simulink model "Enable_Subsystem_Step"  (R2024b)
settings: Solver=FixedStepAuto  StartTime=0.0  StopTime=10.0  FixedStep=0.001  RelTol=1e-3
settings Model: Creator=abdal  LastModifiedBy=abdal

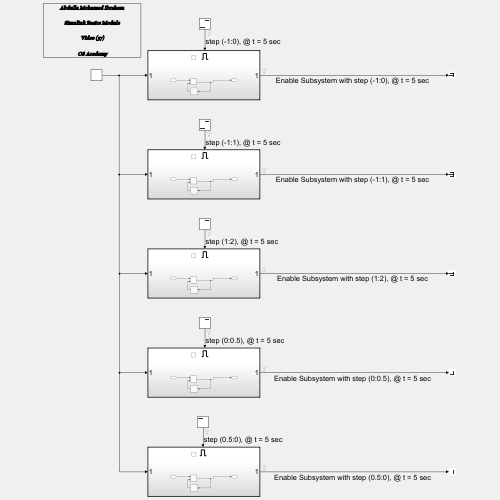
[thumbnail: Simulink's stored preview of the top-level diagram]
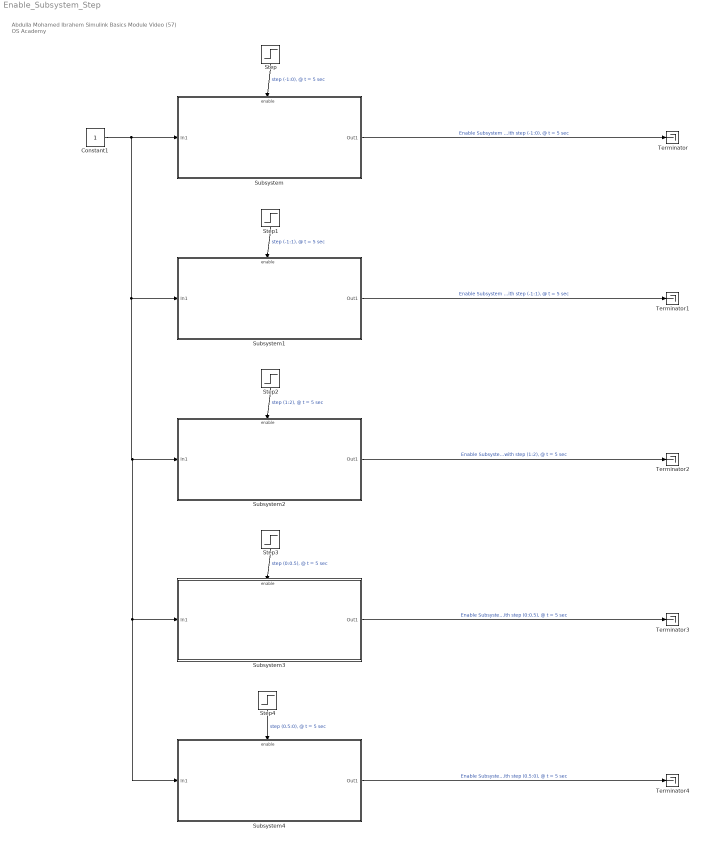
== system Enable_Subsystem_Step ==
  note: Abdulla Mohamed Ibrahem
      | Simulink Basics Module
      | Video (57)
      | OS Academy
  Constant1 : Constant
  Step : Step  Time=5  Before=-1  After=0  SampleTime=0
  Step1 : Step  Time=5  Before=-1  SampleTime=0
  Step2 : Step  Time=5  Before=1  After=2  SampleTime=0
  Step3 : Step  Time=5  After=0.5  SampleTime=0
  Step4 : Step  Time=5  Before=0.5  After=0  SampleTime=0
  Subsystem : Subsystem  TreatAsAtomicUnit=on
  Subsystem1 : Subsystem  TreatAsAtomicUnit=on
  Subsystem2 : Subsystem  TreatAsAtomicUnit=on
  Subsystem3 : Subsystem  TreatAsAtomicUnit=on
  Subsystem4 : Subsystem  TreatAsAtomicUnit=on
  Terminator{,1..4} (5 alike) : Terminator
  wires:
  Subsystem3/1(Out1) -> Terminator3/1  "Enable Subsystem with step (0:0.5), @ t = 5 sec"
  Subsystem2/1(Out1) -> Terminator2/1  "Enable Subsystem with step (1:2), @ t = 5 sec"
  Subsystem1/1(Out1) -> Terminator1/1  "Enable Subsystem with step (-1:1), @ t = 5 sec"
  Step3/1 -> Subsystem3/Enable  "step (0:0.5), @ t = 5 sec"
  Step2/1 -> Subsystem2/Enable  "step (1:2), @ t = 5 sec"
  Step1/1 -> Subsystem1/Enable  "step (-1:1), @ t = 5 sec"
  Subsystem/1(Out1) -> Terminator/1  "Enable Subsystem with step (-1:0), @ t = 5 sec"
  Step/1 -> Subsystem/Enable  "step (-1:0), @ t = 5 sec"
  Step4/1 -> Subsystem4/Enable  "step (0.5:0), @ t = 5 sec"
  Constant1/1 -> Subsystem1/1(In1), Subsystem2/1(In1), Subsystem4/1(In1), Subsystem3/1(In1), Subsystem/1(In1)
  Subsystem4/1(Out1) -> Terminator4/1  "Enable Subsystem with step (0.5:0), @ t = 5 sec"

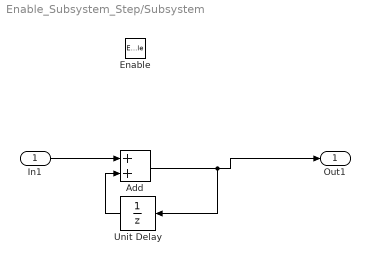
== system Enable_Subsystem_Step/Subsystem ==
  In1 : Inport
  Enable : EnablePort
  Add : Sum
  Unit Delay : UnitDelay  SampleTime=-1  HasFrameUpgradeWarning=on
  Out1 : Outport
  wires:
  Unit Delay/1 -> Add/2
  Add/1 -> Out1/1, Unit Delay/1
  In1/1 -> Add/1

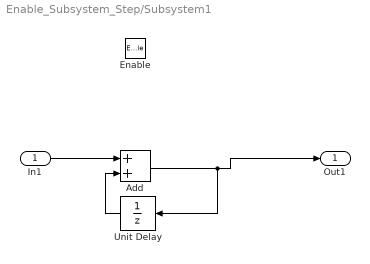
== system Enable_Subsystem_Step/Subsystem1 ==
  In1 : Inport
  Enable : EnablePort
  Add : Sum
  Unit Delay : UnitDelay  SampleTime=-1  HasFrameUpgradeWarning=on
  Out1 : Outport
  wires:
  In1/1 -> Add/1
  Add/1 -> Unit Delay/1, Out1/1
  Unit Delay/1 -> Add/2

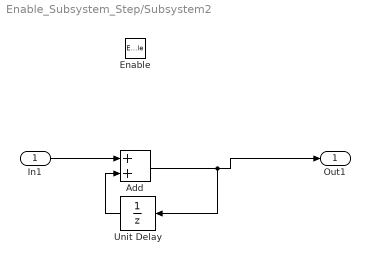
== system Enable_Subsystem_Step/Subsystem2 ==
  In1 : Inport
  Enable : EnablePort
  Add : Sum
  Unit Delay : UnitDelay  SampleTime=-1  HasFrameUpgradeWarning=on
  Out1 : Outport
  wires:
  Unit Delay/1 -> Add/2
  Add/1 -> Out1/1, Unit Delay/1
  In1/1 -> Add/1

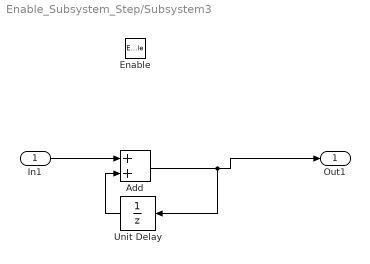
== system Enable_Subsystem_Step/Subsystem3 ==
  In1 : Inport
  Enable : EnablePort  StatesWhenEnabling=reset
  Add : Sum
  Unit Delay : UnitDelay  SampleTime=-1  HasFrameUpgradeWarning=on
  Out1 : Outport
  wires:
  In1/1 -> Add/1
  Add/1 -> Unit Delay/1, Out1/1
  Unit Delay/1 -> Add/2

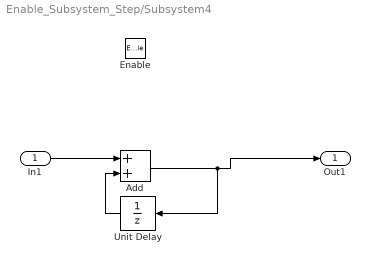
== system Enable_Subsystem_Step/Subsystem4 ==
  In1 : Inport
  Enable : EnablePort  StatesWhenEnabling=reset
  Add : Sum
  Unit Delay : UnitDelay  SampleTime=-1  HasFrameUpgradeWarning=on
  Out1 : Outport
  wires:
  Unit Delay/1 -> Add/2
  Add/1 -> Out1/1, Unit Delay/1
  In1/1 -> Add/1
